simulink model "P1Ej3"  (R2022a)
settings: Solver=VariableStepAuto  StartTime=0.0  StopTime=10.0  RelTol=1e-3
settings Model: Creator=adrian.losada.alvare  LastModifiedBy=Adrian
settings DebuggingCC: UnconnectedInputMsg=warning  UnconnectedOutputMsg=warning  UnconnectedLineMsg=warning
settings RTWCC: DLArmComputeVersion=19.05

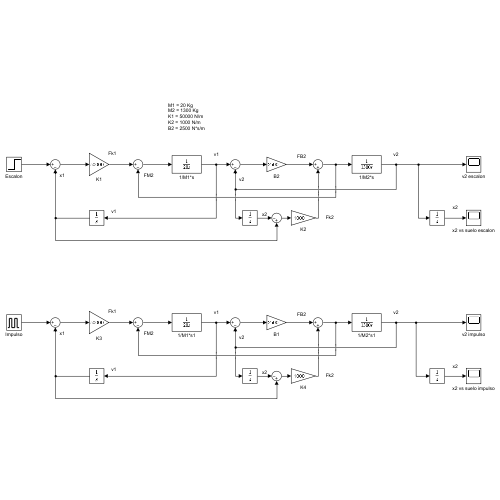
[thumbnail: Simulink's stored preview of the top-level diagram]
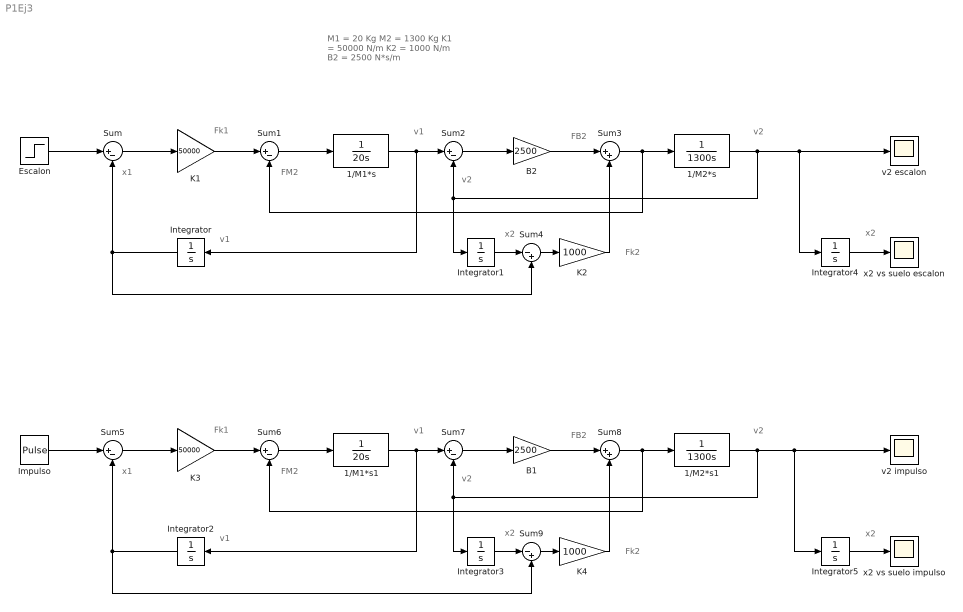
== system P1Ej3 ==
  note: M1 = 20 Kg
      | M2 = 1300 Kg
      | K1 = 50000 N/m
      | K2 = 1000 N/m
      | B2 = 2500 N*s/m
  note: v1
  note: FB2
  note: Fk2
  note: x2
  note: v2
  note: v2
  note: FM2
  note: x1
  note: Fk1
  note: v1
  note: FB2
  note: FM2
  note: v2
  note: v2
  note: v1
  note: v1
  note: x2
  note: x1
  note: Fk2
  note: Fk1
  note: x2
  note: x2
  1/M1*s : TransferFcn  Denominator=[20 0]
  1/M1*s1 : TransferFcn  Denominator=[20 0]
  1/M2*s : TransferFcn  Denominator=[1300 0]
  1/M2*s1 : TransferFcn  Denominator=[1300 0]
  B1 : Gain  Gain=2500
  B2 : Gain  Gain=2500
  Escalon : Step  Time=0  SampleTime=0
  Impulso : DiscretePulseGenerator  PulseType=Time based  Period=10  PulseWidth=5
  Integrator{,1..5} (6 alike) : Integrator
  K1 : Gain  Gain=50000
  K2 : Gain  Gain=1000
  K3 : Gain  Gain=50000
  K4 : Gain  Gain=1000
  Sum{,1..2,5..7} (6 alike) : Sum  Inputs=|+-
  Sum3 : Sum  Inputs=|++
  Sum4 : Sum  Inputs=|-+
  Sum8 : Sum  Inputs=|++
  Sum9 : Sum  Inputs=|-+
  v2 escalon : Scope
  v2 impulso : Scope
  x2 vs suelo escalon : Scope
  x2 vs suelo impulso : Scope
  wires:
  Sum/1 -> K1/1
  K1/1 -> Sum1/1
  Sum1/1 -> 1/M1*s/1
  1/M1*s/1 -> Integrator/1, Sum2/1
  Sum2/1 -> B2/1
  B2/1 -> Sum3/1
  Sum3/1 -> Sum1/2, 1/M2*s/1
  1/M2*s/1 -> Integrator4/1, v2 escalon/1, Sum2/2, Integrator1/1
  Integrator/1 -> Sum4/2, Sum/2
  Integrator1/1 -> Sum4/1
  Sum4/1 -> K2/1
  K2/1 -> Sum3/2
  Escalon/1 -> Sum/1
  K4/1 -> Sum8/2
  Integrator3/1 -> Sum9/1
  1/M2*s1/1 -> Integrator5/1, v2 impulso/1, Sum7/2, Integrator3/1
  Sum5/1 -> K3/1
  Sum7/1 -> B1/1
  K3/1 -> Sum6/1
  1/M1*s1/1 -> Integrator2/1, Sum7/1
  Sum9/1 -> K4/1
  Sum8/1 -> Sum6/2, 1/M2*s1/1
  B1/1 -> Sum8/1
  Sum6/1 -> 1/M1*s1/1
  Integrator2/1 -> Sum9/2, Sum5/2
  Impulso/1 -> Sum5/1
  Integrator4/1 -> x2 vs suelo escalon/1
  Integrator5/1 -> x2 vs suelo impulso/1
